simulink model "SyDdemoPWMOutput"  (Simulink 7.0)
settings: Solver=ode45  StartTime=0.0  StopTime=10.0  RelTol=1e-3
model workspace (MAT data in the model file):
  control_volt : Simulink.Signal (value not decoded)
  battery_volt : Simulink.Signal (value not decoded)
  control_pwm : Simulink.Signal (value not decoded)
  BATTERY_COR_ENA : Simulink.Parameter (value not decoded)
  BATTERY_COR_PWM : Simulink.Parameter (value not decoded)
libraries: simulink x2
settings Model: Creator=Aurelien PROST  LastModifiedBy=Aurelien PROST
settings Model: ModifiedHistory=|
  | <syd:extradata xmlns:syd="http://www.leanpulse.com/schemas/syd/2011/core" owner="LeanPulse" ref="SPEC0002" title="SyD Demo - PWM Output"><syd:version author="Aurélien PROST" date="9 Mar 2011" num="1.0" opt1="" opt2="">This model is referenced by the root demo model "SyDdemo.mdl". It has been created to highlight the generation of multiple documents by following the model dependencies, as enabled by SyD.
  | 
  | (c) LeanPulse 2011</syd:version></syd:extradata>
settings OptimizationCC: InitFltsAndDblsToZero=off
settings DebuggingCC: StrictBusMsg=ErrorLevel1

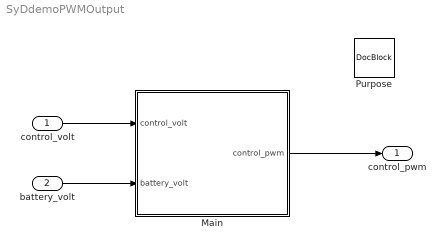
== system SyDdemoPWMOutput ==
  control_volt : Inport
  battery_volt : Inport  Port=2
  Main : Subsystem
  Purpose : simulink/Model-Wide Utilities/DocBlock  SystemSampleTime=-1  DocumentType=RTF
  control_pwm : Outport
  wires:
  control_volt/1 -> Main/1(control_volt)
  battery_volt/1 -> Main/2(battery_volt)
  Main/1(control_pwm) -> control_pwm/1

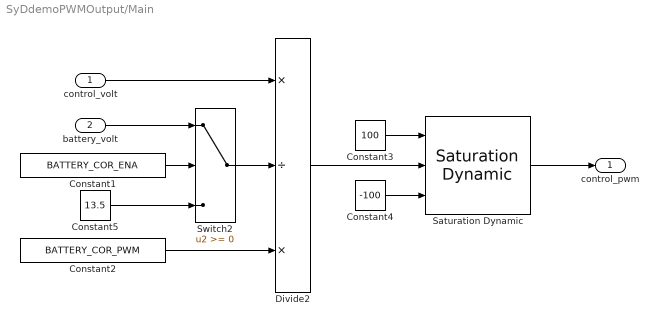
== system SyDdemoPWMOutput/Main ==
  control_volt : Inport
  battery_volt : Inport  Port=2
  Constant1 : Constant  Value=BATTERY_COR_ENA
  Constant2 : Constant  Value=BATTERY_COR_PWM
  Constant3 : Constant  Value=100
  Constant4 : Constant  Value=-100
  Constant5 : Constant  Value=13.5
  Divide2 : Product  Inputs=*/*
  Saturation Dynamic : simulink/Discontinuities/Saturation Dynamic  SystemSampleTime=-1  OutMin=[]  OutMax=[]  OutDataType=fixdt(1, 16)  OutScaling=2^-10  DoSatur=off
  Switch2 : Switch
  control_pwm : Outport
  wires:
  battery_volt/1 -> Switch2/1
  Constant1/1 -> Switch2/2
  Constant5/1 -> Switch2/3
  Switch2/1 -> Divide2/2
  control_volt/1 -> Divide2/1
  Constant2/1 -> Divide2/3
  Divide2/1 -> Saturation Dynamic/2
  Constant4/1 -> Saturation Dynamic/3
  Constant3/1 -> Saturation Dynamic/1
  Saturation Dynamic/1 -> control_pwm/1
